simulink library "velocityAngle_ul"  (R2022a)
settings: Solver=VariableStepAuto  StartTime=0.0  StopTime=10.0  RelTol=1e-3
libraries: gnd2TanRotation_ul x1
settings Model: Creator=mcobb  LastModifiedBy=lhill8
settings SolverCC: AlgebraicLoopSolver=TrustRegion
settings DebuggingCC: UnconnectedInputMsg=warning  UnconnectedOutputMsg=warning  UnconnectedLineMsg=warning  SFMachineParentedDataDiag=warning  ArithmeticOperatorsInVariantConditions=warning
settings SFSimCC: CustomCodeUndefinedFunction=UseInterfaceOnly

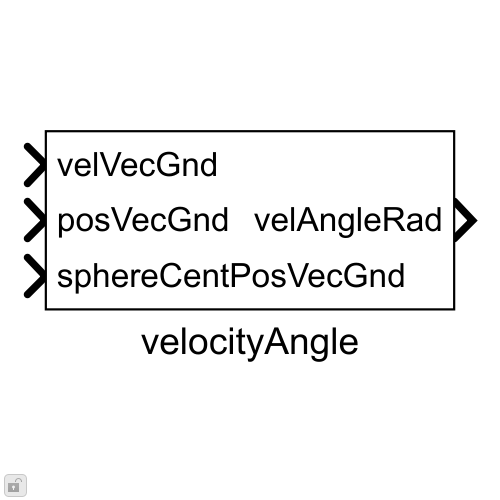
[thumbnail: Simulink's stored preview of the top-level diagram]
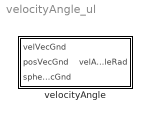
== system velocityAngle_ul ==
  velocityAngle : Subsystem

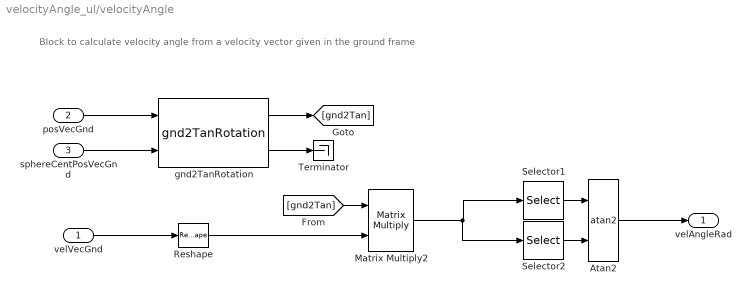
== system velocityAngle_ul/velocityAngle ==
  note: Block to calculate velocity angle from a velocity vector given in the ground frame
  velVecGnd : Inport
  posVecGnd : Inport  Port=2
  sphereCentPosVecGnd : Inport  Port=3
  Atan2 : Trigonometry  Operator=atan2
  Matrix Multiply2 : Product  Multiplication=Matrix(*)
  Reshape : Reshape  OutputDimensionality=Column vector (2-D)
  Selector1 : Selector  InputPortWidth=3  IndexOptions=Index vector (dialog)  Indices=2  OutputSizes=1
  Selector2 : Selector  InputPortWidth=3  IndexOptions=Index vector (dialog)  Indices=1  OutputSizes=1
  Terminator : Terminator
  gnd2TanRotation : gnd2TanRotation_ul/gnd2TanRotation  SystemSampleTime=-1  VariantActivationTime=update diagram  Latency=0  AutoFrameSizeCalculation=off
  velAngleRad : Outport  VectorParamsAs1DForOutWhenUnconnected=off
  wires:
  Matrix Multiply2/1 -> Selector2/1, Selector1/1
  velVecGnd/1 -> Reshape/1
  gnd2TanRotation/2 -> Terminator/1
  posVecGnd/1 -> gnd2TanRotation/1
  sphereCentPosVecGnd/1 -> gnd2TanRotation/2
  gnd2TanRotation/1 -> [gnd2Tan]
  [gnd2Tan] -> Matrix Multiply2/1
  Reshape/1 -> Matrix Multiply2/2
  Selector2/1 -> Atan2/2
  Selector1/1 -> Atan2/1
  Atan2/1 -> velAngleRad/1
